simulink model "untitled"  (R2019b)
settings: Solver=VariableStepAuto  StartTime=0.0  StopTime=1000.0  RelTol=1e-3
libraries: simulink x6
settings Model: Creator=brajm  LastModifiedBy=patti
settings DataIOCC: ReturnWorkspaceOutputs=off
settings DebuggingCC: ArithmeticOperatorsInVariantConditions=warning
settings SFSimCC: CustomCodeUndefinedFunction=UseInterfaceOnly

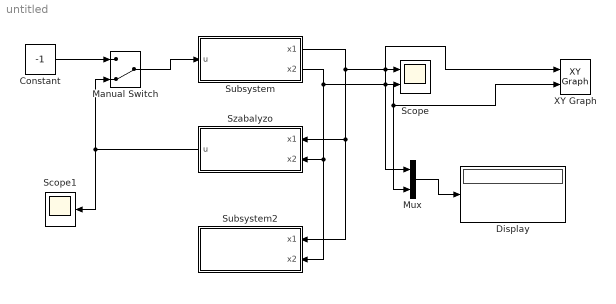
== system untitled ==
  Constant : Constant  Value=-1
  Display : Display
  Manual Switch : ManualSwitch  CurrentSetting=0
  Mux : Mux  Inputs=2
  Scope : Scope  NumInputPorts=2
  Scope1 : Scope
  Subsystem : Subsystem  mask{x0=[20;12]}
  Subsystem2 : Subsystem
  Szabalyzo : Subsystem
  XY Graph : simulink/Sinks/XY Graph  xmin=-100  xmax=100  ymin=-100  ymax=100  st=0.01
  wires:
  Subsystem/1(x1) -> Szabalyzo/1(x1), Subsystem2/1(x1), Mux/1, Scope/1, XY Graph/1
  Constant/1 -> Manual Switch/1
  Manual Switch/1 -> Subsystem/1(u)
  Mux/1 -> Display/1
  Subsystem/2(x2) -> Subsystem2/2(x2), Szabalyzo/2(x2), Mux/2, XY Graph/2, Scope/2
  Szabalyzo/1("u ") -> Scope1/1, Manual Switch/2

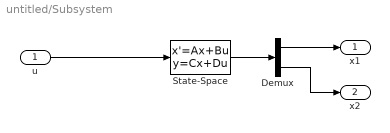
== system untitled/Subsystem ==
  u : Inport
  Demux : Demux  Outputs=2
  State-Space : StateSpace  A=[0 1;0 0]  B=[0;1]  C=[1 0;0 1]  D=[0;0]  InitialCondition=x0
  x1 : Outport  VectorParamsAs1DForOutWhenUnconnected=off
  x2 : Outport  Port=2  VectorParamsAs1DForOutWhenUnconnected=off
  wires:
  u/1 -> State-Space/1
  State-Space/1 -> Demux/1
  Demux/1 -> x1/1
  Demux/2 -> x2/1

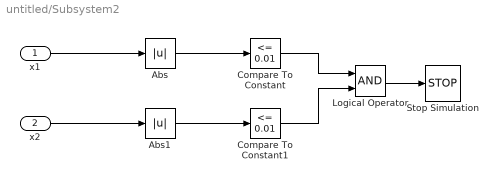
== system untitled/Subsystem2 ==
  x1 : Inport
  x2 : Inport  Port=2
  Abs : Abs
  Abs1 : Abs
  Compare To Constant : simulink/Logic and Bit Operations/Compare To Constant  relop=<=  const=0.01  OutDataTypeStr=boolean
  Compare To Constant1 : simulink/Logic and Bit Operations/Compare To Constant  relop=<=  const=0.01  OutDataTypeStr=boolean
  Logical Operator : Logic  AllPortsSameDT=off  OutDataTypeStr=boolean
  Stop Simulation : Stop
  wires:
  x2/1 -> Abs1/1
  x1/1 -> Abs/1
  Abs1/1 -> Compare To Constant1/1
  Abs/1 -> Compare To Constant/1
  Compare To Constant1/1 -> Logical Operator/2
  Compare To Constant/1 -> Logical Operator/1
  Logical Operator/1 -> Stop Simulation/1

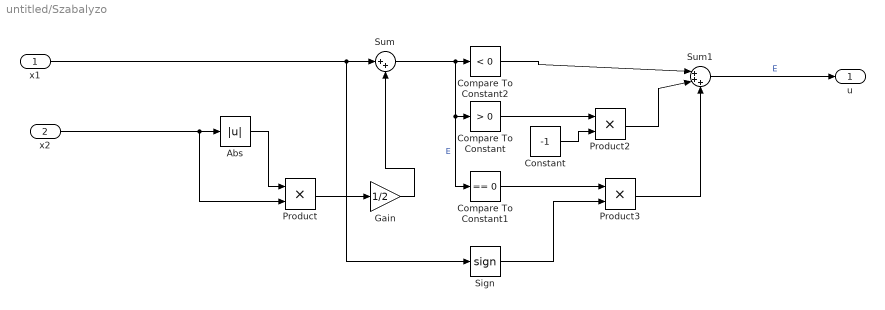
== system untitled/Szabalyzo ==
  x1 : Inport
  x2 : Inport  Port=2
  Abs : Abs
  Compare To Constant : simulink/Logic and Bit Operations/Compare To Constant  relop=>  const=0  OutDataTypeStr=boolean
  Compare To Constant1 : simulink/Logic and Bit Operations/Compare To Constant  relop===  const=0  OutDataTypeStr=boolean
  Compare To Constant2 : simulink/Logic and Bit Operations/Compare To Constant  relop=<  const=0  OutDataTypeStr=boolean
  Constant : Constant  Value=-1
  Gain : Gain  Gain=1/2
  Product : Product
  Product2 : Product
  Product3 : Product
  Sign : Signum
  Sum : Sum  Inputs=|++
  Sum1 : Sum  Inputs=|+++
  "u " : Outport  VectorParamsAs1DForOutWhenUnconnected=off
  wires:
  Compare To Constant2/1 -> Sum1/1
  x2/1 -> Product/2, Abs/1
  Product3/1 -> Sum1/3
  Compare To Constant/1 -> Product2/1
  Compare To Constant1/1 -> Product3/1
  Sum/1 -> Compare To Constant/1, Compare To Constant1/1, Compare To Constant2/1  "E"
  Constant/1 -> Product2/2
  Gain/1 -> Sum/2
  Sign/1 -> Product3/2
  Abs/1 -> Product/1
  Sum1/1 -> "u "/1  "E"
  x1/1 -> Sum/1, Sign/1
  Product/1 -> Gain/1
  Product2/1 -> Sum1/2
